simulink library "NC_MDL"  (R2015a)
settings: Solver=ode45  StartTime=0.0  StopTime=10.0  RelTol=1e-3
undefined symbols (not defined in the file or in its folder): NC
libraries: simulink x1
settings Model: Creator=Andrew  LastModifiedBy=Andrew

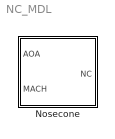
== system NC_MDL ==
  Nosecone : Subsystem  mask{NC=NC}
      mask prompts: NC "INPUTS"

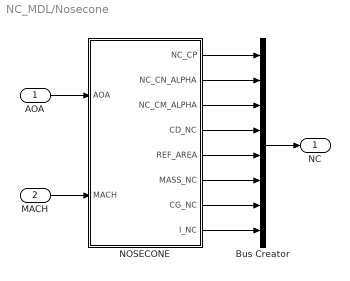
== system NC_MDL/Nosecone ==
  AOA : Inport
  MACH : Inport  Port=2
  Bus Creator : BusCreator  Inputs=8
  NOSECONE : Subsystem
  NC : Outport
  wires:
  Bus Creator/1 -> NC/1
  MACH/1 -> NOSECONE/2(MACH)
  AOA/1 -> NOSECONE/1(AOA)
  NOSECONE/4(CD_NC) -> Bus Creator/4
  NOSECONE/6(MASS_NC) -> Bus Creator/6
  NOSECONE/5(REF_AREA) -> Bus Creator/5
  NOSECONE/7(CG_NC) -> Bus Creator/7
  NOSECONE/2(NC_CN_ALPHA) -> Bus Creator/2
  NOSECONE/1(NC_CP) -> Bus Creator/1
  NOSECONE/8(I_NC) -> Bus Creator/8
  NOSECONE/3(NC_CM_ALPHA) -> Bus Creator/3

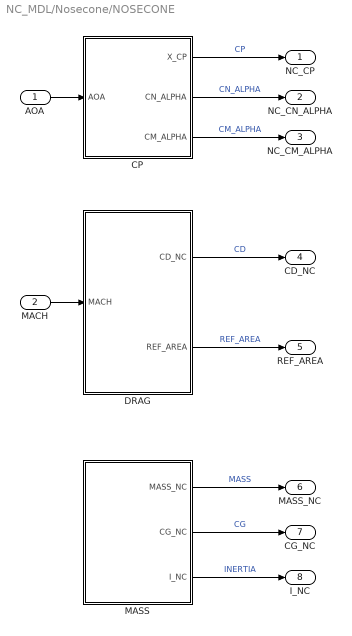
== system NC_MDL/Nosecone/NOSECONE ==
  AOA : Inport
  MACH : Inport  Port=2
  CP : Subsystem
  DRAG : Subsystem
  MASS : Subsystem
  NC_CP : Outport
  NC_CN_ALPHA : Outport  Port=2
  NC_CM_ALPHA : Outport  Port=3
  CD_NC : Outport  Port=4
  REF_AREA : Outport  Port=5
  MASS_NC : Outport  Port=6
  CG_NC : Outport  Port=7
  I_NC : Outport  Port=8
  wires:
  CP/1(X_CP) -> NC_CP/1  "CP"
  CP/2(CN_ALPHA) -> NC_CN_ALPHA/1  "CN_ALPHA"
  DRAG/1(CD_NC) -> CD_NC/1  "CD"
  DRAG/2(REF_AREA) -> REF_AREA/1  "REF_AREA"
  AOA/1 -> CP/1(AOA)
  MACH/1 -> DRAG/1(MACH)
  CP/3(CM_ALPHA) -> NC_CM_ALPHA/1  "CM_ALPHA"
  MASS/1(MASS_NC) -> MASS_NC/1  "MASS"
  MASS/2(CG_NC) -> CG_NC/1  "CG"
  MASS/3(I_NC) -> I_NC/1  "INERTIA"

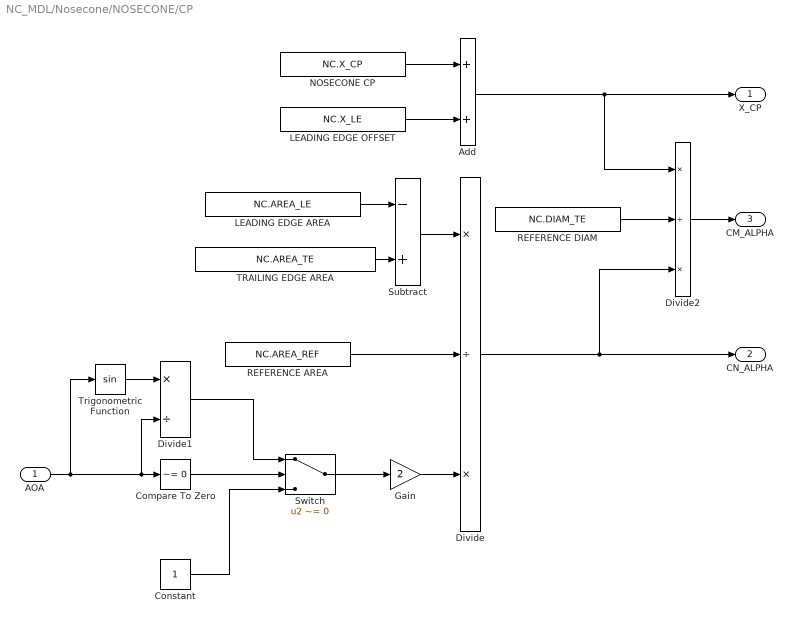
== system NC_MDL/Nosecone/NOSECONE/CP ==
  AOA : Inport
  Add : Sum
  Compare To Zero : simulink/Logic and Bit Operations/Compare To Zero  relop=~=  OutDataTypeStr=boolean
  Constant : Constant
  Divide : Product  Inputs=*/*
  Divide1 : Product  Inputs=*/
  Divide2 : Product  Inputs=*/*
  Gain : Gain  Gain=2
  LEADING EDGE AREA : FromWorkspace  VariableName=NC.AREA_LE
  LEADING EDGE OFFSET : FromWorkspace  VariableName=NC.X_LE
  NOSECONE CP : FromWorkspace  VariableName=NC.X_CP
  REFERENCE AREA : FromWorkspace  VariableName=NC.AREA_REF
  REFERENCE DIAM : FromWorkspace  VariableName=NC.DIAM_TE
  Subtract : Sum  Inputs=-+
  Switch : Switch  Criteria=u2 ~= 0
  TRAILING EDGE AREA : FromWorkspace  VariableName=NC.AREA_TE
  Trigonometric Function : Trigonometry  OutputSignalType=real
  X_CP : Outport
  CN_ALPHA : Outport  Port=2
  CM_ALPHA : Outport  Port=3
  wires:
  Divide1/1 -> Switch/1
  Trigonometric Function/1 -> Divide1/1
  LEADING EDGE AREA/1 -> Subtract/1
  TRAILING EDGE AREA/1 -> Subtract/2
  Subtract/1 -> Divide/1
  AOA/1 -> Compare To Zero/1, Divide1/2, Trigonometric Function/1
  Constant/1 -> Switch/3
  Compare To Zero/1 -> Switch/2
  Switch/1 -> Gain/1
  REFERENCE AREA/1 -> Divide/2
  Divide/1 -> Divide2/3, CN_ALPHA/1
  Add/1 -> Divide2/1, X_CP/1
  LEADING EDGE OFFSET/1 -> Add/2
  NOSECONE CP/1 -> Add/1
  Gain/1 -> Divide/3
  Divide2/1 -> CM_ALPHA/1
  REFERENCE DIAM/1 -> Divide2/2

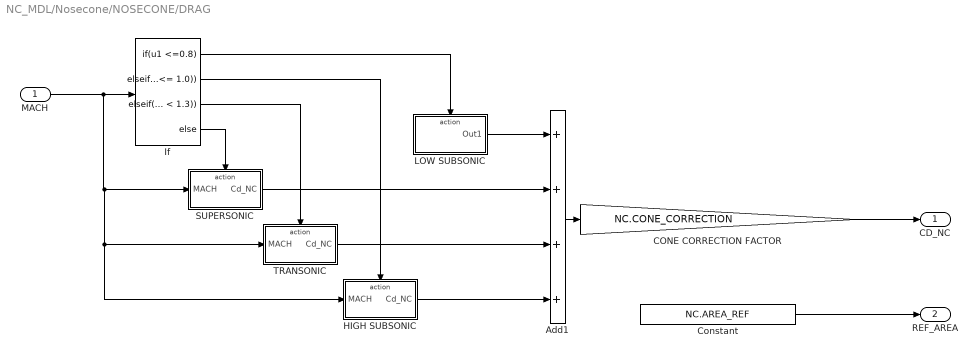
== system NC_MDL/Nosecone/NOSECONE/DRAG ==
  MACH : Inport
  Add1 : Sum  Inputs=++++
  CONE CORRECTION FACTOR : Gain  Gain=NC.CONE_CORRECTION
  Constant : Constant  Value=NC.AREA_REF
  HIGH SUBSONIC : Subsystem  TreatAsAtomicUnit=on
  If : If  IfExpression=u1 <=0.8  ElseIfExpressions=(u1 > 0.8) & (u1 <= 1.0), (u1 > 1) & (u1 < 1.3)
  LOW SUBSONIC : Subsystem  TreatAsAtomicUnit=on
  SUPERSONIC : Subsystem  TreatAsAtomicUnit=on
  TRANSONIC : Subsystem  TreatAsAtomicUnit=on
  CD_NC : Outport
  REF_AREA : Outport  Port=2
  wires:
  Constant/1 -> REF_AREA/1
  MACH/1 -> If/1, SUPERSONIC/1(MACH), TRANSONIC/1(MACH), HIGH SUBSONIC/1(MACH)
  If/4 -> SUPERSONIC/Action
  If/2 -> HIGH SUBSONIC/Action
  Add1/1 -> CONE CORRECTION FACTOR/1
  SUPERSONIC/1(Cd_NC) -> Add1/2
  If/1 -> LOW SUBSONIC/Action
  If/3 -> TRANSONIC/Action
  TRANSONIC/1(Cd_NC) -> Add1/3
  HIGH SUBSONIC/1(Cd_NC) -> Add1/4
  LOW SUBSONIC/1(Out1) -> Add1/1
  CONE CORRECTION FACTOR/1 -> CD_NC/1

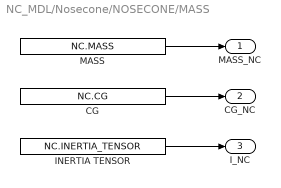
== system NC_MDL/Nosecone/NOSECONE/MASS ==
  CG : Constant  Value=NC.CG
  INERTIA TENSOR : Constant  Value=NC.INERTIA_TENSOR
  MASS : Constant  Value=NC.MASS
  MASS_NC : Outport
  CG_NC : Outport  Port=2
  I_NC : Outport  Port=3
  wires:
  INERTIA TENSOR/1 -> I_NC/1
  MASS/1 -> MASS_NC/1
  CG/1 -> CG_NC/1

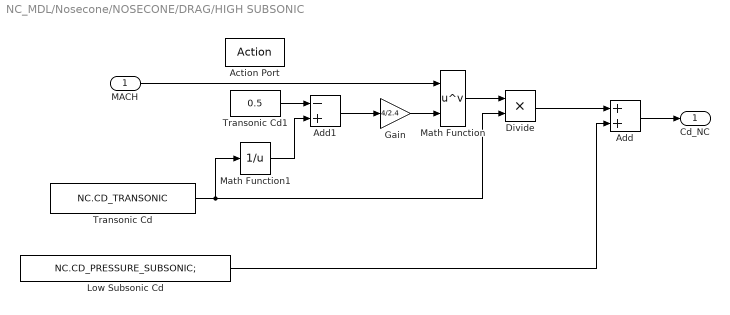
== system NC_MDL/Nosecone/NOSECONE/DRAG/HIGH SUBSONIC ==
  MACH : Inport
  Action Port : ActionPort
  Add : Sum
  Add1 : Sum  Inputs=-+
  Divide : Product  Inputs=**
  Gain : Gain  Gain=4/2.4
  Low Subsonic Cd : Constant  Value=NC.CD_PRESSURE_SUBSONIC;
  Math Function : Math  Operator=pow  SaturateOnIntegerOverflow=on
  Math Function1 : Math  Operator=reciprocal  SaturateOnIntegerOverflow=on
  Transonic Cd : Constant  Value=NC.CD_TRANSONIC
  Transonic Cd1 : Constant  Value=0.5
  Cd_NC : Outport
  wires:
  Gain/1 -> Math Function/2
  Add1/1 -> Gain/1
  Transonic Cd1/1 -> Add1/1
  Math Function1/1 -> Add1/2
  Transonic Cd/1 -> Divide/2, Math Function1/1
  Low Subsonic Cd/1 -> Add/2
  Math Function/1 -> Divide/1
  MACH/1 -> Math Function/1
  Divide/1 -> Add/1
  Add/1 -> Cd_NC/1

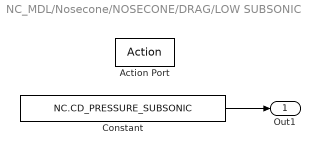
== system NC_MDL/Nosecone/NOSECONE/DRAG/LOW SUBSONIC ==
  Action Port : ActionPort
  Constant : Constant  Value=NC.CD_PRESSURE_SUBSONIC
  Out1 : Outport
  wires:
  Constant/1 -> Out1/1

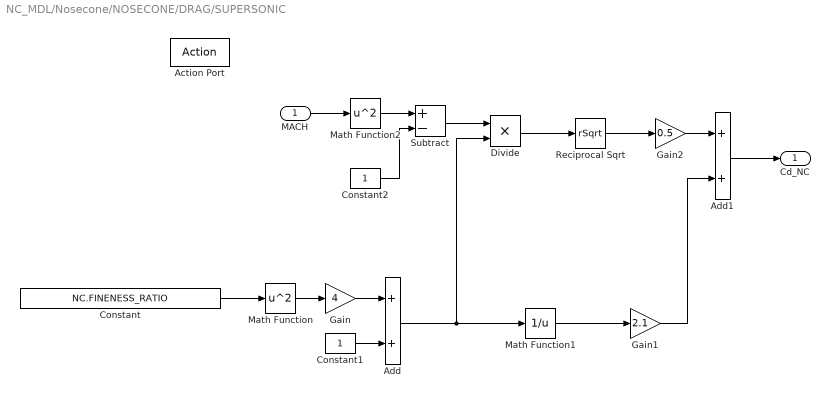
== system NC_MDL/Nosecone/NOSECONE/DRAG/SUPERSONIC ==
  MACH : Inport
  Action Port : ActionPort
  Add : Sum
  Add1 : Sum
  Constant : Constant  Value=NC.FINENESS_RATIO
  Constant1 : Constant
  Constant2 : Constant
  Divide : Product  Inputs=**
  Gain : Gain  Gain=4
  Gain1 : Gain  Gain=2.1
  Gain2 : Gain  Gain=0.5
  Math Function : Math  Operator=square  SaturateOnIntegerOverflow=on
  Math Function1 : Math  Operator=reciprocal  SaturateOnIntegerOverflow=on
  Math Function2 : Math  Operator=square  SaturateOnIntegerOverflow=on
  Reciprocal Sqrt : Sqrt  Operator=rSqrt  SaturateOnIntegerOverflow=on
  Subtract : Sum  Inputs=+-
  Cd_NC : Outport
  wires:
  Constant2/1 -> Subtract/2
  Math Function2/1 -> Subtract/1
  MACH/1 -> Math Function2/1
  Subtract/1 -> Divide/1
  Divide/1 -> Reciprocal Sqrt/1
  Reciprocal Sqrt/1 -> Gain2/1
  Gain2/1 -> Add1/1
  Add/1 -> Math Function1/1, Divide/2
  Math Function1/1 -> Gain1/1
  Gain1/1 -> Add1/2
  Add1/1 -> Cd_NC/1
  Constant1/1 -> Add/2
  Gain/1 -> Add/1
  Math Function/1 -> Gain/1
  Constant/1 -> Math Function/1

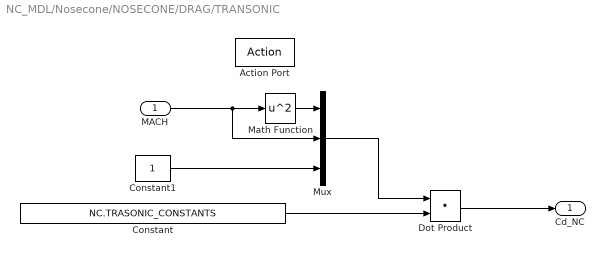
== system NC_MDL/Nosecone/NOSECONE/DRAG/TRANSONIC ==
  MACH : Inport
  Action Port : ActionPort
  Constant : Constant  Value=NC.TRASONIC_CONSTANTS
  Constant1 : Constant
  Dot Product : DotProduct  InputSameDT=on  OutDataTypeStr=Inherit: Inherit via internal rule
  Math Function : Math  Operator=square  SaturateOnIntegerOverflow=on
  Mux : Mux  Inputs=3
  Cd_NC : Outport
  wires:
  Dot Product/1 -> Cd_NC/1
  Math Function/1 -> Mux/1
  Constant/1 -> Dot Product/2
  Mux/1 -> Dot Product/1
  Constant1/1 -> Mux/3
  MACH/1 -> Math Function/1, Mux/2
